simulink model "Conversor_Angulo_Voltagem"  (R2022b)
settings: Solver=VariableStepAuto  StartTime=0.0  StopTime=10.0  RelTol=1e-3
libraries: fl_lib x13, nesl_utility x4, ee_lib x1
settings Model: Creator=matheusassis  LastModifiedBy=matheusassis

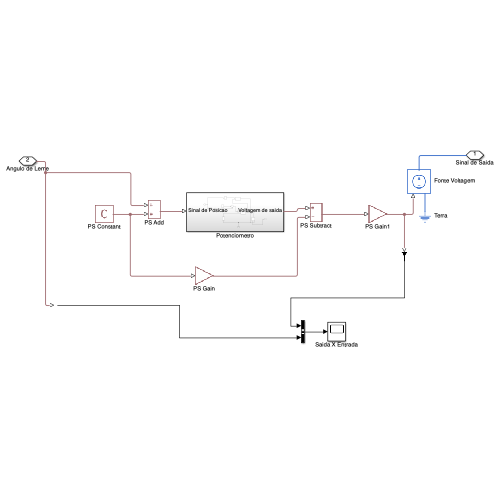
[thumbnail: Simulink's stored preview of the top-level diagram]
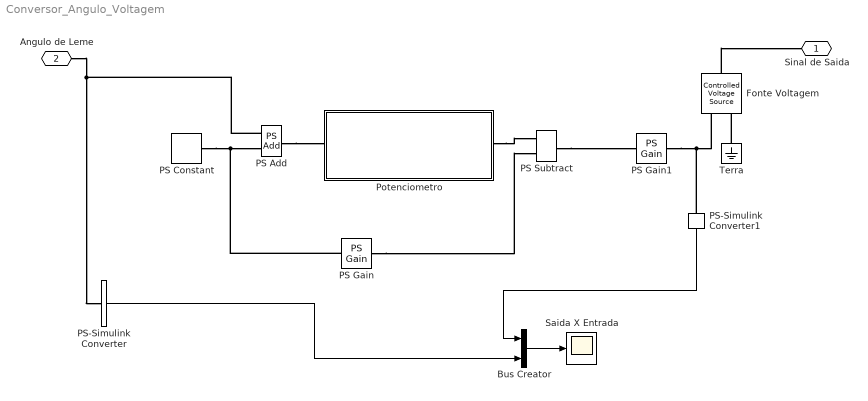
== system Conversor_Angulo_Voltagem ==
  Bus Creator : BusCreator  Inputs=2
  Fonte Voltagem : fl_lib/Electrical/Electrical Sources/Controlled Voltage Source
  PS Add : fl_lib/Physical Signals/Functions/PS Add
  PS Constant : fl_lib/Physical Signals/Sources/PS Constant  constant=1
  PS Gain : fl_lib/Physical Signals/Functions/PS Gain  gain=1
  PS Gain1 : fl_lib/Physical Signals/Functions/PS Gain  gain=1
  PS Subtract : fl_lib/Physical Signals/Functions/PS Subtract
  PS-Simulink Converter : nesl_utility/PS-Simulink Converter  PhysicalDomain=network_engine_domain  SubClassName=ps_output  LeftPortType=input  RightPortType=output  PseudoPeriodic=off  Frequencies=[]  VectorFormat=inherit  Unit=inherit  AffineConversion=off
  PS-Simulink Converter1 : nesl_utility/PS-Simulink Converter  PhysicalDomain=network_engine_domain  SubClassName=ps_output  LeftPortType=input  RightPortType=output  PseudoPeriodic=off  Frequencies=[]  VectorFormat=inherit  Unit=inherit  AffineConversion=off
  Potenciometro : Subsystem
  Saida X Entrada : Scope
  Terra : fl_lib/Electrical/Electrical Elements/Electrical Reference
  Sinal de Saida : PMIOPort  Side=Left
  Angulo de Leme : PMIOPort  Port=2  Side=Left
  wires:
  PS-Simulink Converter/1 -> Bus Creator/2
  PS-Simulink Converter1/1 -> Bus Creator/1
  Bus Creator/1 -> Saida X Entrada/1
  connections:
  Angulo de Leme/RConn1 -- PS Add/LConn1 -- PS-Simulink Converter/LConn1
  PS Constant/RConn1 -- PS Gain/LConn1 -- PS Add/LConn2
  PS Gain/RConn1 -- PS Subtract/LConn2
  PS Subtract/RConn1 -- PS Gain1/LConn1
  PS Gain1/RConn1 -- PS-Simulink Converter1/LConn1 -- Fonte Voltagem/RConn1
  Terra/LConn1 -- Fonte Voltagem/RConn2
  Fonte Voltagem/LConn1 -- Sinal de Saida/RConn1
  Potenciometro/RConn1 -- PS Subtract/LConn1
  PS Add/RConn1 -- Potenciometro/LConn1

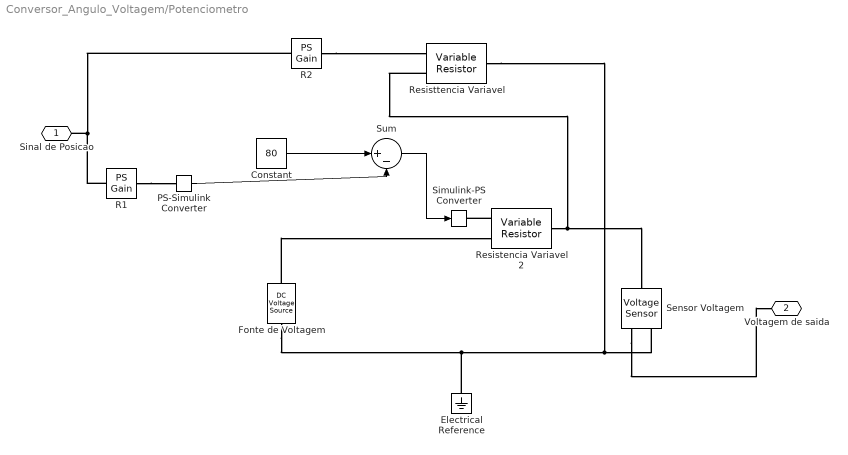
== system Conversor_Angulo_Voltagem/Potenciometro ==
  " Fonte de Voltagem" : ee_lib/Additional Components/SPICE Sources/DC Voltage Source  DC=10 V
  Constant : Constant  Value=80
  Electrical Reference : fl_lib/Electrical/Electrical Elements/Electrical Reference
  PS-Simulink Converter : nesl_utility/PS-Simulink Converter  PhysicalDomain=network_engine_domain  SubClassName=ps_output  LeftPortType=input  RightPortType=output  PseudoPeriodic=off  Frequencies=[]  VectorFormat=inherit  Unit=inherit  AffineConversion=off
  R1 : fl_lib/Physical Signals/Functions/PS Gain  gain=1
  R2 : fl_lib/Physical Signals/Functions/PS Gain  gain=1
  Resistencia Variavel 2 : fl_lib/Electrical/Electrical Elements/Variable Resistor  Rmin=0 Ohm  i_specify=off  i_priority=None  i=0 A  i_nominal_specify=off  i_nominal_unit=A  i_nominal_value=1  v_specify=off  v_priority=None  v=0 V  v_nominal_specify=off  v_nominal_unit=V  v_nominal_value=1
  Resisttencia Variavel : fl_lib/Electrical/Electrical Elements/Variable Resistor  Rmin=0 Ohm  i_specify=off  i_priority=None  i=0 A  i_nominal_specify=off  i_nominal_unit=A  i_nominal_value=1  v_specify=off  v_priority=None  v=0 V  v_nominal_specify=off  v_nominal_unit=V  v_nominal_value=1
  "Sensor Voltagem " : fl_lib/Electrical/Electrical Sensors/Voltage Sensor
  Simulink-PS Converter : nesl_utility/Simulink-PS Converter  PhysicalDomain=network_engine_domain  SubClassName=ps_input  LeftPortType=input  RightPortType=output  PseudoPeriodic=off  Frequencies=[]  NoiseDistribution=none  NoiseParameters=[]  Unit=1  AffineConversion=off  FilteringAndDerivatives=provide  SimscapeFilterOrder=1  InputFilterTimeConstant=0.001  UdotUserProvided=0
  Sum : Sum  Inputs=|+-
  Sinal de Posicao : PMIOPort  Side=Left
  Voltagem de saida : PMIOPort  Port=2  Side=Right
  wires:
  Constant/1 -> Sum/1
  PS-Simulink Converter/1 -> Sum/2
  Sum/1 -> Simulink-PS Converter/1
  connections:
  Sinal de Posicao/RConn1 -- R1/LConn1 -- R2/LConn1
  "Sensor Voltagem "/RConn2 -- Resisttencia Variavel/RConn1 -- Electrical Reference/LConn1 -- " Fonte de Voltagem"/RConn1
  Resisttencia Variavel/LConn2 -- Resistencia Variavel 2/RConn1 -- "Sensor Voltagem "/LConn1
  R1/RConn1 -- PS-Simulink Converter/LConn1
  Resistencia Variavel 2/LConn1 -- Simulink-PS Converter/RConn1
  " Fonte de Voltagem"/LConn1 -- Resistencia Variavel 2/LConn2
  "Sensor Voltagem "/RConn1 -- Voltagem de saida/RConn1
  R2/RConn1 -- Resisttencia Variavel/LConn1
